simulink model "OL_BSC"  (R2015b)
settings: Solver=FixedStepDiscrete  StartTime=0.0  StopTime=final_time  FixedStep=bsck_stepSize  RelTol=1e-3
libraries: simulink x1
settings Model: Creator=nctzv8  LastModifiedBy=nctzv8
settings ConfigSet: Description=OpenECU configuration set for code generation under RTW-EC.
settings SolverCC: PositivePriorityOrder=on
settings DataIOCC: SaveFormat=Array  SignalLoggingSaveFormat=ModelDataLogs
settings OptimizationCC: DefaultParameterBehavior=Inlined  InlineInvariantSignals=on  ExpressionDepthLimit=2147483647  StateBitsets=on  DataBitsets=on  ZeroExternalMemoryAtStartup=off  ZeroInternalMemoryAtStartup=off  NoFixptDivByZeroProtection=on  EfficientFloat2IntCast=on  OptimizeModelRefInitCode=on  LifeSpan=1
settings DebuggingCC: SaveWithParameterizedLinksMsg=none  UnderspecifiedInitializationDetection=Classic  MergeDetectMultiDrivingBlocksExec=none  SignalResolutionControl=TryResolveAllWithWarning  MultiTaskDSMMsg=warning  MultiTaskCondExecSysMsg=none  SingleTaskRateTransMsg=error  CheckMatrixSingularityMsg=warning  VectorMatrixConversionMsg=warning  FcnCallInpInsideContextMsg=UseLocalSettings  SignalLabelMismatchMsg=warning  StateNameClashWarn=warning
settings HardwareCC: ProdBitPerPointer=32  ProdLargestAtomicInteger=Long  ProdLargestAtomicFloat=Double  ProdEndianess=BigEndian  ProdWordSize=32  ProdHWDeviceType=Freescale->32-bit PowerPC  TargetIntDivRoundTo=Zero  TargetEndianess=BigEndian  TargetHWDeviceType=Freescale->32-bit PowerPC  ProdEqTarget=off
settings RTWCC: SystemTargetFile=openecu_ert.tlc  MakeCommand=make_rtw optimized_floating_point=1  TemplateMakefile=openecu_ert_r2015b_64.tmf  Description=OpenECU Platform Target (ERT, optimised floating-point code)  RetainRTWFile=on  IncludeHyperlinkInReport=on
settings CodeAppCC: ForceParamTrailComments=on  IgnoreCustomStorageClasses=off  SimulinkDataObjDesc=on  CustomSymbolStrType=$N$R$M  InsertBlockDesc=on  InternalIdentifier=Classic
settings STFCustomTargetCC: TargetLibSuffix=.a  GenerateSampleERTMain=on  ModelReferenceCompliant=off  ConcurrentExecutionCompliant=off  IncludeMdlTerminateFcn=off  GeneratePreprocessorConditionals=Use local settings  CombineOutputUpdateFcns=on  IncludeFileDelimiter=UseQuote  ERTCustomFileBanners=on  SupportContinuousTime=off  MATLABClassNameForMDSCustomization=Simulink.SoftwareTarget.ERTCustomization  CPPClassGenCompliant=off  GRTInterface=off  SystemTargetFile=openecu_ert.tlc
settings ERTTargetCC: GenerateSampleERTMain=on  ModelReferenceCompliant=off  ParMdlRefBuildCompliant=off  CompOptLevelCompliant=off  ConcurrentExecutionCompliant=off  IncludeMdlTerminateFcn=off  ERTFirstTimeCompliant=off  IncludeFileDelimiter=UseQuote  SupportNonInlinedSFcns=on  ModelStepFunctionPrototypeControlCompliant=off  CPPClassGenCompliant=off  UseToolchainInfoCompliant=off  ExtModeMexFile=noextcomm  InlinedParameterPlacement=NonHierarchical  ERTSrcFileBannerTemplate=oe_code_c_template.cgt  ERTHdrFileBannerTemplate=oe_code_h_template.cgt  ERTDataSrcFileTemplate=oe_data_c_template.cgt  ERTDataHdrFileTemplate=oe_data_h_template.cgt  ERTCustomFileTemplate=example_file_process.tlc  GlobalDataDefinition=InSeparateSourceFile  GlobalDataReference=InSeparateHeaderFile  EnableUserReplacementTypes=on

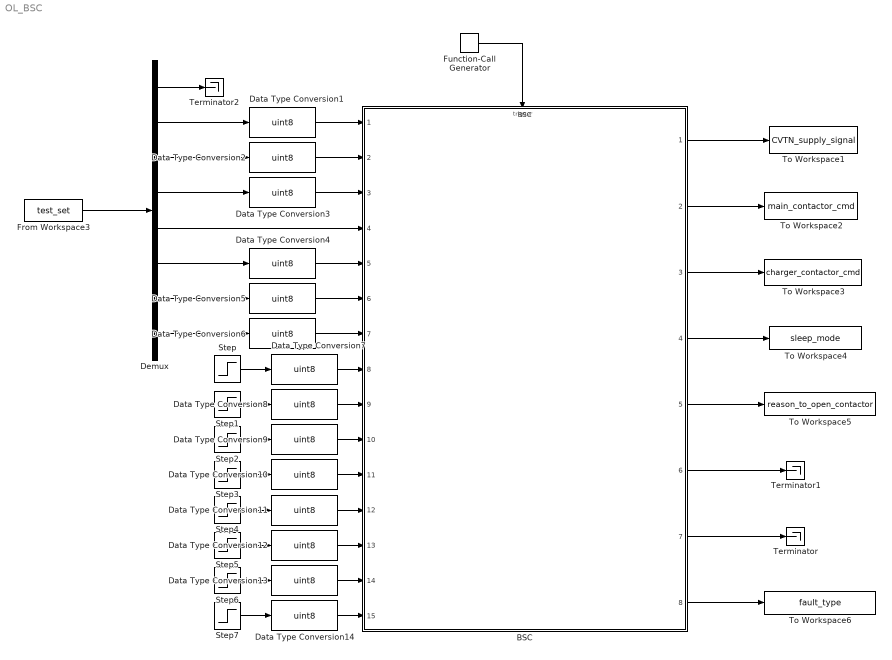
== system OL_BSC ==
  BSC : ModelReference  ModelNameDialog=BSC.slx  SimulationMode=Normal  ModelReferenceVersion=1.220  CopyOfModelName=BSC.slx  TriggerPortName=Trigger  TriggerPortTriggerType=function-call  TriggerPortStatesWhenEnabling=held
  Data Type Conversion{1..14} (14 alike) : DataTypeConversion  OutDataTypeStr=uint8
  Demux : Demux  Outputs=8
  From Workspace3 : FromWorkspace  VariableName=test_set  SampleTime=0
  Function-Call Generator : simulink/Ports & Subsystems/Function-Call Generator  sample_time=bsck_stepSize  numberOfIterations=1
  Step{,1..7} (8 alike) : Step  Time=0  After=0  VectorParams1D=off
  Terminator : Terminator
  Terminator1 : Terminator
  Terminator2 : Terminator
  To Workspace1 : ToWorkspace  VariableName=CVTN_supply_signal  SaveFormat=Timeseries  SampleTime=-1
  To Workspace2 : ToWorkspace  VariableName=main_contactor_cmd  SaveFormat=Timeseries  SampleTime=-1
  To Workspace3 : ToWorkspace  VariableName=charger_contactor_cmd  SaveFormat=Timeseries  SampleTime=-1
  To Workspace4 : ToWorkspace  VariableName=sleep_mode  SaveFormat=Timeseries  SampleTime=-1
  To Workspace5 : ToWorkspace  VariableName=reason_to_open_contactor  SaveFormat=Timeseries  SampleTime=-1
  To Workspace6 : ToWorkspace  VariableName=fault_type  SaveFormat=Timeseries  SampleTime=-1
  wires:
  Demux/2 -> Data Type Conversion1/1
  Demux/3 -> Data Type Conversion2/1
  Demux/4 -> Data Type Conversion3/1
  Demux/6 -> Data Type Conversion4/1
  Demux/7 -> Data Type Conversion5/1
  Demux/8 -> Data Type Conversion6/1
  BSC/7 -> Terminator/1
  From Workspace3/1 -> Demux/1
  BSC/1 -> To Workspace1/1
  BSC/2 -> To Workspace2/1
  BSC/3 -> To Workspace3/1
  BSC/4 -> To Workspace4/1
  BSC/5 -> To Workspace5/1
  BSC/6 -> Terminator1/1
  BSC/8 -> To Workspace6/1
  Function-Call Generator/1 -> BSC/Trigger
  Data Type Conversion1/1 -> BSC/1
  Data Type Conversion2/1 -> BSC/2
  Data Type Conversion3/1 -> BSC/3
  Demux/5 -> BSC/4
  Data Type Conversion4/1 -> BSC/5
  Data Type Conversion5/1 -> BSC/6
  Data Type Conversion6/1 -> BSC/7
  Demux/1 -> Terminator2/1
  Step/1 -> Data Type Conversion7/1
  Step2/1 -> Data Type Conversion9/1
  Step1/1 -> Data Type Conversion8/1
  Step3/1 -> Data Type Conversion10/1
  Step4/1 -> Data Type Conversion11/1
  Step6/1 -> Data Type Conversion13/1
  Step7/1 -> Data Type Conversion14/1
  Step5/1 -> Data Type Conversion12/1
  Data Type Conversion7/1 -> BSC/8
  Data Type Conversion8/1 -> BSC/9
  Data Type Conversion9/1 -> BSC/10
  Data Type Conversion10/1 -> BSC/11
  Data Type Conversion11/1 -> BSC/12
  Data Type Conversion12/1 -> BSC/13
  Data Type Conversion13/1 -> BSC/14
  Data Type Conversion14/1 -> BSC/15
